simulink model "SC_Test_ROS"  (R2023a)
settings: Solver=VariableStepAuto  StartTime=0.0  StopTime=inf  RelTol=1e-3
libraries: robotlib x4
settings Model: Creator=gptp  LastModifiedBy=gptp

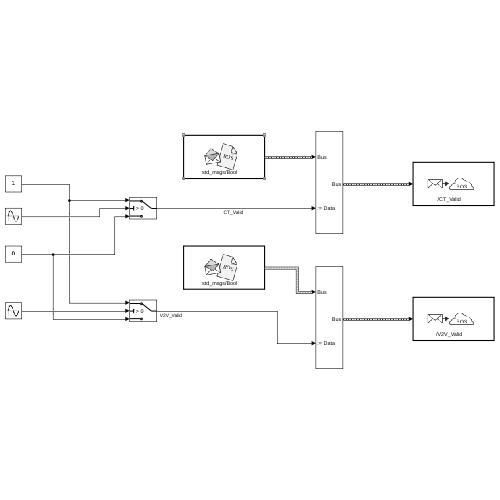
[thumbnail: Simulink's stored preview of the top-level diagram]
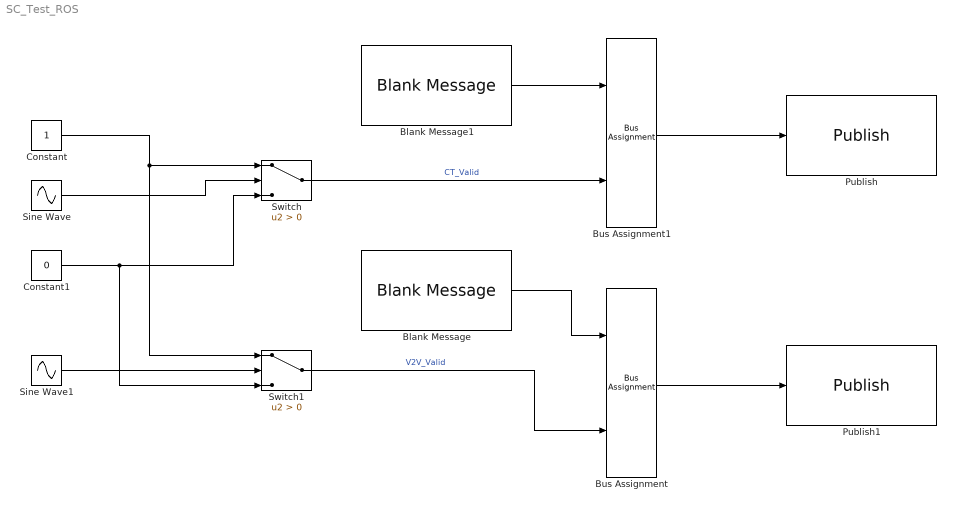
== system SC_Test_ROS ==
  Blank Message : robotlib/Blank Message  messageClass=Message  entityType=std_msgs/Bool  messageType=std_msgs/Bool  SampleTime=inf  legacyBusStruct=off
  Blank Message1 : robotlib/Blank Message  messageClass=Message  entityType=std_msgs/Bool  messageType=std_msgs/Bool  SampleTime=inf  legacyBusStruct=off
  Bus Assignment : BusAssignment  AssignedSignals=Data
  Bus Assignment1 : BusAssignment  AssignedSignals=Data
  Constant : Constant  OutDataTypeStr=boolean
  Constant1 : Constant  Value=0  OutDataTypeStr=boolean
  Publish : robotlib/Publish  topicSource=Specify your own  topic=/CT_Valid  messageType=std_msgs/Bool  legacyBusStruct=off  messageQueueLength=1
  Publish1 : robotlib/Publish  topicSource=Specify your own  topic=/V2V_Valid  messageType=std_msgs/Bool  legacyBusStruct=off  messageQueueLength=1
  Sine Wave : Sin  SampleTime=0
  Sine Wave1 : Sin  Phase=pi/2  SampleTime=0
  Switch : Switch  Criteria=u2 > Threshold  OutDataTypeStr=boolean  SaturateOnIntegerOverflow=off  InputSameDT=off
  Switch1 : Switch  Criteria=u2 > Threshold  OutDataTypeStr=boolean  SaturateOnIntegerOverflow=off  InputSameDT=off
  wires:
  Sine Wave/1 -> Switch/2
  Constant1/1 -> Switch1/3, Switch/3
  Constant/1 -> Switch1/1, Switch/1
  Sine Wave1/1 -> Switch1/2
  Switch1/1 -> Bus Assignment/2  "V2V_Valid"
  Blank Message/1 -> Bus Assignment/1
  Switch/1 -> Bus Assignment1/2  "CT_Valid"
  Blank Message1/1 -> Bus Assignment1/1
  Bus Assignment1/1 -> Publish/1
  Bus Assignment/1 -> Publish1/1
